simulink model "Biomech_Project_LQR_cleanup"  (R2017a)
settings: Solver=ode45  StartTime=0.0  StopTime=10  MaxStep=1e-3  RelTol=1e-4  AbsTol=1e-6  EnableMultiTasking=on
values from neighbouring files (symbols this model uses):
  g = 9.81    [Biomech_Project_LQR_param.mat]
  K = [0.0235570993622  0.453677279991  -0.304744102928; 0.280809210373  -0.335573491599  -0.504535045423]    [Biomech_Project_LQR_param.mat]    (also in QRABK_LQR_controller.mat)
  L = 0.2    [Biomech_Project_LQR_param.mat]
  l0 = 0.2    [Biomech_Project_LQR_param.mat]
  m = 6    [Biomech_Project_LQR_param.mat]
  x0 = []    [AnimQUAD.m]    (also in Biomech_Project_LQR_param.mat = 0)
  xrb0 = 0.130612869685    [Biomech_Project_LQR_param.mat]
  xrf0 = -0.273446372372    [Biomech_Project_LQR_param.mat]
  y0 = 1    [Biomech_Project_LQR_param.mat]
  yrb0 = 0.187577786922    [Biomech_Project_LQR_param.mat]
  yrf0 = 0.186025886331    [Biomech_Project_LQR_param.mat]
libraries: simulink_extras x4
settings Model: Creator=hgeyer  LastModifiedBy=shawn
settings DataIOCC: SaveFormat=Array  SignalLoggingSaveFormat=ModelDataLogs
settings OptimizationCC: ExpressionDepthLimit=2147483647  LifeSpan=inf
settings DebuggingCC: UnderspecifiedInitializationDetection=Classic  MergeDetectMultiDrivingBlocksExec=none  SolverPrmCheckMsg=warning  FcnCallInpInsideContextMsg=warning  AllowSymbolicDim=off  StateNameClashWarn=warning  SFUnexpectedBacktrackingDiag=warning  SFNoUnconditionalDefaultTransitionDiag=warning  SFExecutionAtInitializationDiag=none
settings HardwareCC: ProdBitPerPointer=32  ProdBitPerSizeT=32  ProdBitPerPtrDiffT=32  ProdLargestAtomicFloat=None  ProdIntDivRoundTo=Undefined  ProdEndianess=Unspecified  ProdWordSize=32  ProdHWDeviceType=32-bit Generic
settings ModelReferenceCC: PropagateSignalLabelsOutOfModel=off
settings GRTTargetCC: TargetLangStandard=C89/C90 (ANSI)  GeneratePreprocessorConditionals=Disable all
settings ConfigComp: CovMetricSettings=dw  CovHtmlReporting=on  CovSaveCumulativeToWorkspaceVar=on  CovSaveSingleToWorkspaceVar=on  CovExternalEMLEnable=off

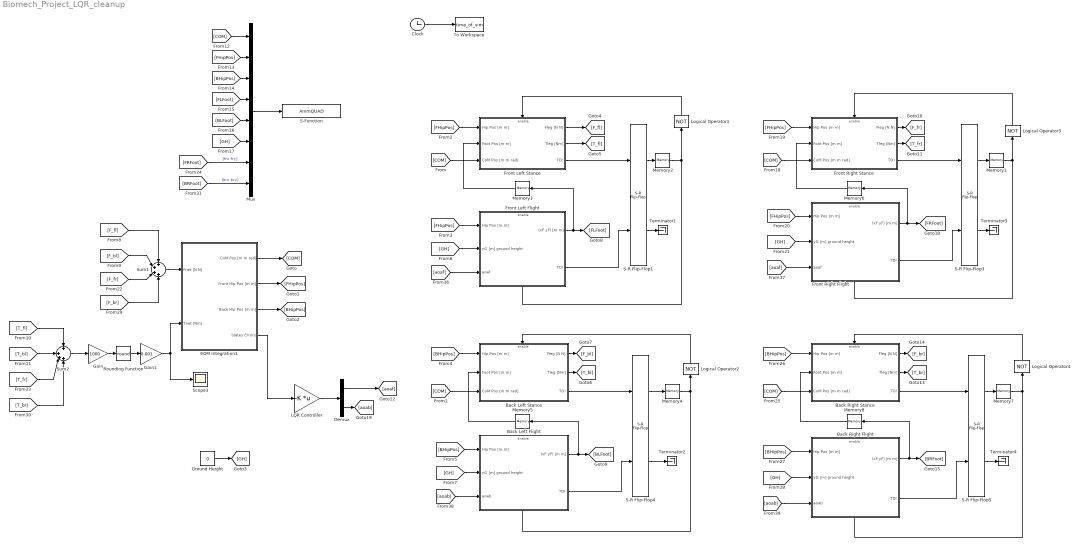
== system Biomech_Project_LQR_cleanup ==
  Back Left Flight : Subsystem
  Back Left Stance : Subsystem
  Back Right Flight : Subsystem
  Back Right Stance : Subsystem
  Clock : Clock
      settings: Decimation=100
  Demux : Demux  Outputs=2
  EOM Integration1 : Subsystem
  Front Left Flight : Subsystem
  Front Left Stance : Subsystem
  Front Right Flight : Subsystem
  Front Right Stance : Subsystem
  Gain : Gain  Gain=1000
  Gain1 : Gain  Gain=0.001
  Ground Height : Constant  Value=0
  LQR Controller : Gain  Gain=-K  Multiplication=Matrix(K*u)
  Logical Operator{1..4} (4 alike) : Logic  Operator=NOT  AllPortsSameDT=off  OutDataTypeStr=boolean
  Memory{1..2,4,7} (4 alike) : Memory  X0=1
  Memory3 : Memory  X0=[(x0 - xrf0) (y0 - yrf0) ]
  Memory5 : Memory  X0=[(x0 - xrb0) (y0 - yrb0)]
  Memory6 : Memory  X0=[(x0 - xrf0) (y0 - yrf0) ]
  Memory8 : Memory  X0=[(x0 - xrb0) (y0 - yrb0)]
  Mux : Mux  Inputs=8
  Rounding Function : Rounding  Operator=round
  S-Function : S-Function  FunctionName=AnimQUAD  Parameters=0.005  SFunctionDeploymentMode=off  EnableBusSupport=off
  S-R Flip-Flop{1,3..5} (4 alike) : simulink_extras/Flip Flops/S-R Flip-Flop  initial_condition=1
  Scope3 : Scope
  Sum1 : Sum  Inputs=++++
  Sum2 : Sum  Inputs=+|+++
  Terminator{1..4} (4 alike) : Terminator
  To Workspace : ToWorkspace  VariableName=time_of_sim  SampleTime=-1
      settings: MaxDataPoints=1
  wires:
  S-R Flip-Flop1/1 -> Memory2/1
  Memory2/1 -> Front Left Flight/Enable, Logical Operator1/1
  Logical Operator1/1 -> Front Left Stance/Enable
  S-R Flip-Flop1/2 -> Terminator1/1
  Front Left Flight/1((xF yF) [m m]) -> Memory3/1, [FLFoot]
  Memory3/1 -> Front Left Stance/2(Foot Pos [m m])
  Back Left Stance/3(TO!) -> S-R Flip-Flop4/1
  S-R Flip-Flop4/1 -> Memory4/1
  Back Left Flight/2(TD!) -> S-R Flip-Flop4/2
  Memory4/1 -> Back Left Flight/Enable, Logical Operator2/1
  Logical Operator2/1 -> Back Left Stance/Enable
  S-R Flip-Flop4/2 -> Terminator2/1
  [GH] -> Back Left Flight/2(yG [m] ground height)
  Back Left Flight/1((xF yF) [m m]) -> [BLFoot], Memory5/1
  Memory5/1 -> Back Left Stance/2(Foot Pos [m m])
  Ground Height/1 -> [GH]
  [GH] -> Front Left Flight/2(yG [m] ground height)
  Front Left Stance/1(Fleg [N N]) -> [F_fl]
  Front Left Stance/2(Tleg [Nm]) -> [T_fl]
  Back Left Stance/1(Fleg [N N]) -> [F_bl]
  Back Left Stance/2(Tleg [Nm]) -> [T_bl]
  [F_fl] -> Sum1/1
  [F_bl] -> Sum1/2
  [T_fl] -> Sum2/1
  [T_bl] -> Sum2/2
  Sum1/1 -> EOM Integration1/1(Fnet [N N])
  EOM Integration1/1(CoM Pos [m m rad]) -> [COM]
  EOM Integration1/2(Front Hip Pos [m m]) -> [FHipPos]
  EOM Integration1/3(Back Hip Pos [m m]) -> [BHipPos]
  [FHipPos] -> Front Left Stance/1(Hip Pos [m m])
  [FHipPos] -> Front Left Flight/1(Hip Pos [m m])
  [BHipPos] -> Back Left Stance/1(Hip Pos [m m])
  [BHipPos] -> Back Left Flight/1(Hip Pos [m m])
  [COM] -> Front Left Stance/3(CoM Pos [m m rad])
  [COM] -> Back Left Stance/3(CoM Pos [m m rad])
  Sum2/1 -> Gain/1
  Gain1/1 -> Scope3/1, EOM Integration1/2(Tnet [Nm])
  Gain/1 -> Rounding Function/1
  Rounding Function/1 -> Gain1/1
  Mux/1 -> S-Function/1
  [COM] -> Mux/1
  [FHipPos] -> Mux/2
  [BHipPos] -> Mux/3
  [FLFoot] -> Mux/4
  [BLFoot] -> Mux/5
  [GH] -> Mux/6
  [FRFoot] -> Mux/7  "[frx fry]"
  [BRFoot] -> Mux/8  "[brx bry]"
  S-R Flip-Flop3/1 -> Memory1/1
  Memory1/1 -> Front Right Flight/Enable, Logical Operator3/1
  Logical Operator3/1 -> Front Right Stance/Enable
  S-R Flip-Flop3/2 -> Terminator3/1
  Front Right Flight/1((xF yF) [m m]) -> [FRFoot], Memory6/1
  Memory6/1 -> Front Right Stance/2(Foot Pos [m m])
  [GH] -> Front Right Flight/2(yG [m] ground height)
  Front Right Stance/1(Fleg [N N]) -> [F_fr]
  Front Right Stance/2(Tleg [Nm]) -> [T_fr]
  [FHipPos] -> Front Right Stance/1(Hip Pos [m m])
  [FHipPos] -> Front Right Flight/1(Hip Pos [m m])
  [COM] -> Front Right Stance/3(CoM Pos [m m rad])
  [F_fr] -> Sum1/3
  [T_fr] -> Sum2/3
  Back Right Stance/3(TO!) -> S-R Flip-Flop5/1
  S-R Flip-Flop5/1 -> Memory7/1
  Back Right Flight/2(TD!) -> S-R Flip-Flop5/2
  Memory7/1 -> Back Right Flight/Enable, Logical Operator4/1
  Logical Operator4/1 -> Back Right Stance/Enable
  S-R Flip-Flop5/2 -> Terminator4/1
  [GH] -> Back Right Flight/2(yG [m] ground height)
  Back Right Flight/1((xF yF) [m m]) -> [BRFoot], Memory8/1
  Memory8/1 -> Back Right Stance/2(Foot Pos [m m])
  Back Right Stance/1(Fleg [N N]) -> [F_br]
  Back Right Stance/2(Tleg [Nm]) -> [T_br]
  [BHipPos] -> Back Right Stance/1(Hip Pos [m m])
  [BHipPos] -> Back Right Flight/1(Hip Pos [m m])
  [COM] -> Back Right Stance/3(CoM Pos [m m rad])
  [F_br] -> Sum1/4
  [T_br] -> Sum2/4
  Clock/1 -> To Workspace/1
  Front Right Stance/3(TO!) -> S-R Flip-Flop3/1
  Front Right Flight/2(TD!) -> S-R Flip-Flop3/2
  Front Left Stance/3(TO!) -> S-R Flip-Flop1/1
  Front Left Flight/2(TD!) -> S-R Flip-Flop1/2
  EOM Integration1/4(States Errors) -> LQR Controller/1
  LQR Controller/1 -> Demux/1
  Demux/1 -> [aoaf]
  Demux/2 -> [aoab]
  [aoaf] -> Front Left Flight/3("aoaf ")
  [aoaf] -> Front Right Flight/3("aoaf ")
  [aoab] -> Back Left Flight/3(aoab)
  [aoab] -> Back Right Flight/3(aoab)

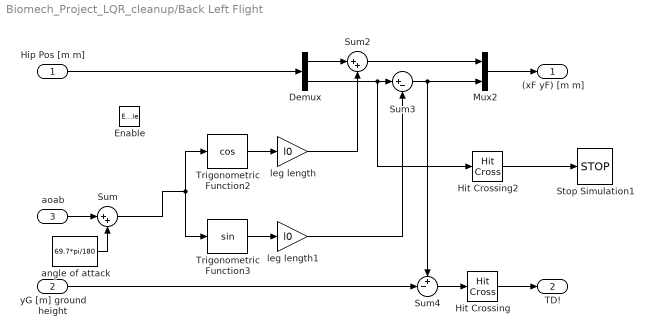
== system Biomech_Project_LQR_cleanup/Back Left Flight ==
  Hip Pos [m m] : Inport
  yG [m] ground height : Inport  Port=2
  aoab : Inport  Port=3
  Enable : EnablePort  StatesWhenEnabling=reset
  Demux : Demux  Outputs=2
  Hit Crossing : HitCross  HitCrossingDirection=falling
  Hit Crossing2 : HitCross  HitCrossingOffset=-1  HitCrossingDirection=falling
  Mux2 : Mux  Inputs=2
  Stop Simulation1 : Stop
  Sum : Sum  Inputs=|++
  Sum2 : Sum  Inputs=|++
  Sum3 : Sum  Inputs=|+-
  Sum4 : Sum  Inputs=+-|
  Trigonometric Function2 : Trigonometry  Operator=cos
  Trigonometric Function3 : Trigonometry
  angle of attack : Constant  Value=69.7*pi/180
  leg length : Gain  Gain=l0
  leg length1 : Gain  Gain=l0
  (xF yF) [m m] : Outport  InitialOutput=[0 0]
      settings: AttributesFormatString=%<OutputWhenDisabled>
  TD! : Outport  Port=2  OutputWhenDisabled=reset  InitialOutput=0
      settings: AttributesFormatString=%<OutputWhenDisabled>
  wires:
  Demux/2 -> Hit Crossing2/1, Sum3/1
  Demux/1 -> Sum2/1
  Sum/1 -> Trigonometric Function3/1, Trigonometric Function2/1
  Trigonometric Function2/1 -> leg length/1
  Trigonometric Function3/1 -> leg length1/1
  Hip Pos [m m]/1 -> Demux/1
  leg length/1 -> Sum2/2
  leg length1/1 -> Sum3/2
  Sum3/1 -> Mux2/2, Sum4/1
  Sum2/1 -> Mux2/1
  Mux2/1 -> (xF yF) [m m]/1
  yG [m] ground height/1 -> Sum4/2
  Sum4/1 -> Hit Crossing/1
  Hit Crossing2/1 -> Stop Simulation1/1
  Hit Crossing/1 -> TD!/1
  aoab/1 -> Sum/1
  angle of attack/1 -> Sum/2

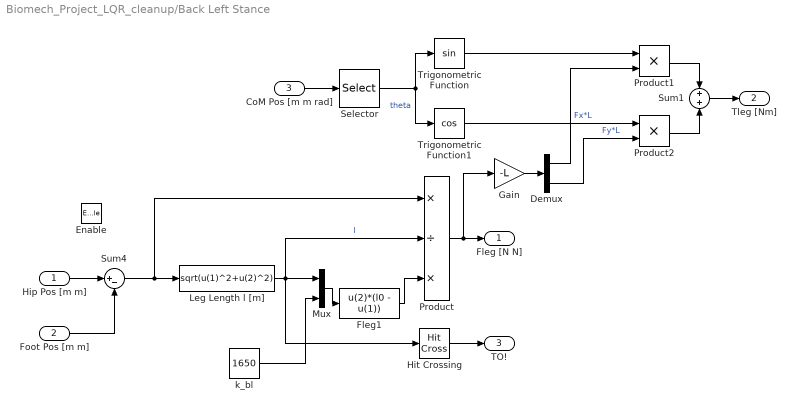
== system Biomech_Project_LQR_cleanup/Back Left Stance ==
  Hip Pos [m m] : Inport
  Foot Pos [m m] : Inport  Port=2
  CoM Pos [m m rad] : Inport  Port=3
  Enable : EnablePort  StatesWhenEnabling=reset
  Demux : Demux  Outputs=2
  Fleg1 : Fcn  Expr=u(2)*(l0 - u(1))
  Gain : Gain  Gain=-L
  Hit Crossing : HitCross  HitCrossingOffset=l0  HitCrossingDirection=rising
  Leg Length l [m] : Fcn  Expr=sqrt(u(1)^2+u(2)^2)
  Mux : Mux  Inputs=2
  Product : Product  Inputs=*/*
  Product1 : Product
  Product2 : Product
  Selector : Selector  InputPortWidth=3  IndexOptions=Index vector (dialog)  Indices=[3]  OutputSizes=1
  Sum1 : Sum  Inputs=+|+
  Sum4 : Sum  Inputs=|+-
  Trigonometric Function : Trigonometry
  Trigonometric Function1 : Trigonometry  Operator=cos
  k_bl : Constant  Value=1650
  Fleg [N N] : Outport  OutputWhenDisabled=reset  InitialOutput=[0 0]
      settings: AttributesFormatString=%<OutputWhenDisabled>
  Tleg [Nm] : Outport  Port=2  OutputWhenDisabled=reset  InitialOutput=[0]
      settings: AttributesFormatString=%<OutputWhenDisabled>
  TO! : Outport  Port=3  OutputWhenDisabled=reset  InitialOutput=[0]
      settings: AttributesFormatString=%<OutputWhenDisabled>
  wires:
  Sum1/1 -> Tleg [Nm]/1
  Product1/1 -> Sum1/1
  Product2/1 -> Sum1/2
  Gain/1 -> Demux/1
  Demux/2 -> Product2/2  "Fy*L"
  Demux/1 -> Product1/2  "Fx*L"
  Trigonometric Function/1 -> Product1/1
  Trigonometric Function1/1 -> Product2/1
  Selector/1 -> Trigonometric Function/1, Trigonometric Function1/1  "theta"
  CoM Pos [m m rad]/1 -> Selector/1
  Foot Pos [m m]/1 -> Sum4/2
  Hip Pos [m m]/1 -> Sum4/1
  Hit Crossing/1 -> TO!/1
  Product/1 -> Fleg [N N]/1, Gain/1
  Fleg1/1 -> Product/3
  Leg Length l [m]/1 -> Hit Crossing/1, Mux/1, Product/2  "l"
  Sum4/1 -> Leg Length l [m]/1, Product/1
  Mux/1 -> Fleg1/1
  k_bl/1 -> Mux/2

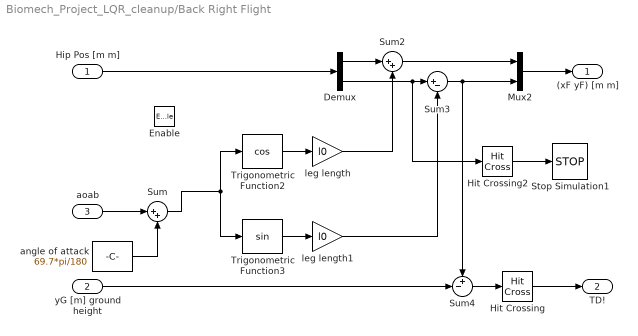
== system Biomech_Project_LQR_cleanup/Back Right Flight ==
  Hip Pos [m m] : Inport
  yG [m] ground height : Inport  Port=2
  aoab : Inport  Port=3
  Enable : EnablePort  StatesWhenEnabling=reset
  Demux : Demux  Outputs=2
  Hit Crossing : HitCross  HitCrossingDirection=falling
  Hit Crossing2 : HitCross  HitCrossingOffset=-1  HitCrossingDirection=falling
  Mux2 : Mux  Inputs=2
  Stop Simulation1 : Stop
  Sum : Sum  Inputs=|++
  Sum2 : Sum  Inputs=|++
  Sum3 : Sum  Inputs=|+-
  Sum4 : Sum  Inputs=+-|
  Trigonometric Function2 : Trigonometry  Operator=cos
  Trigonometric Function3 : Trigonometry
  angle of attack : Constant  Value=69.7*pi/180
  leg length : Gain  Gain=l0
  leg length1 : Gain  Gain=l0
  (xF yF) [m m] : Outport  InitialOutput=[0 0]
      settings: AttributesFormatString=%<OutputWhenDisabled>
  TD! : Outport  Port=2  OutputWhenDisabled=reset  InitialOutput=0
      settings: AttributesFormatString=%<OutputWhenDisabled>
  wires:
  Sum4/1 -> Hit Crossing/1
  yG [m] ground height/1 -> Sum4/2
  Mux2/1 -> (xF yF) [m m]/1
  Sum2/1 -> Mux2/1
  Sum3/1 -> Sum4/1, Mux2/2
  leg length1/1 -> Sum3/2
  leg length/1 -> Sum2/2
  Hip Pos [m m]/1 -> Demux/1
  Trigonometric Function3/1 -> leg length1/1
  Trigonometric Function2/1 -> leg length/1
  Sum/1 -> Trigonometric Function2/1, Trigonometric Function3/1
  Demux/1 -> Sum2/1
  Demux/2 -> Hit Crossing2/1, Sum3/1
  Hit Crossing2/1 -> Stop Simulation1/1
  aoab/1 -> Sum/1
  angle of attack/1 -> Sum/2
  Hit Crossing/1 -> TD!/1

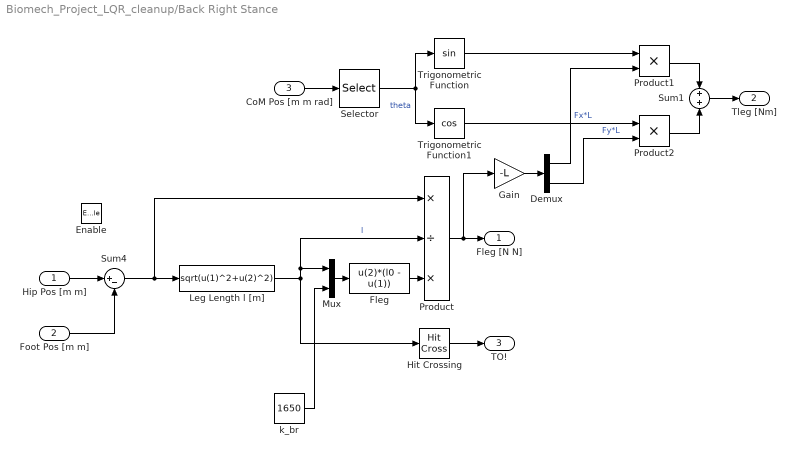
== system Biomech_Project_LQR_cleanup/Back Right Stance ==
  Hip Pos [m m] : Inport
  Foot Pos [m m] : Inport  Port=2
  CoM Pos [m m rad] : Inport  Port=3
  Enable : EnablePort  StatesWhenEnabling=reset
  Demux : Demux  Outputs=2
  Fleg : Fcn  Expr=u(2)*(l0 - u(1))
  Gain : Gain  Gain=-L
  Hit Crossing : HitCross  HitCrossingOffset=l0  HitCrossingDirection=rising
  Leg Length l [m] : Fcn  Expr=sqrt(u(1)^2+u(2)^2)
  Mux : Mux  Inputs=2
  Product : Product  Inputs=*/*
  Product1 : Product
  Product2 : Product
  Selector : Selector  InputPortWidth=3  IndexOptions=Index vector (dialog)  Indices=[3]  OutputSizes=1
  Sum1 : Sum  Inputs=+|+
  Sum4 : Sum  Inputs=|+-
  Trigonometric Function : Trigonometry
  Trigonometric Function1 : Trigonometry  Operator=cos
  k_br : Constant  Value=1650
  Fleg [N N] : Outport  OutputWhenDisabled=reset  InitialOutput=[0 0]
      settings: AttributesFormatString=%<OutputWhenDisabled>
  Tleg [Nm] : Outport  Port=2  OutputWhenDisabled=reset  InitialOutput=[0]
      settings: AttributesFormatString=%<OutputWhenDisabled>
  TO! : Outport  Port=3  OutputWhenDisabled=reset  InitialOutput=[0]
      settings: AttributesFormatString=%<OutputWhenDisabled>
  wires:
  Sum1/1 -> Tleg [Nm]/1
  Product1/1 -> Sum1/1
  Product2/1 -> Sum1/2
  Gain/1 -> Demux/1
  Demux/2 -> Product2/2  "Fy*L"
  Demux/1 -> Product1/2  "Fx*L"
  Trigonometric Function/1 -> Product1/1
  Trigonometric Function1/1 -> Product2/1
  Selector/1 -> Trigonometric Function/1, Trigonometric Function1/1  "theta"
  CoM Pos [m m rad]/1 -> Selector/1
  Foot Pos [m m]/1 -> Sum4/2
  Hip Pos [m m]/1 -> Sum4/1
  Hit Crossing/1 -> TO!/1
  Product/1 -> Fleg [N N]/1, Gain/1
  Fleg/1 -> Product/3
  Leg Length l [m]/1 -> Mux/1, Product/2, Hit Crossing/1  "l"
  Sum4/1 -> Leg Length l [m]/1, Product/1
  Mux/1 -> Fleg/1
  k_br/1 -> Mux/2

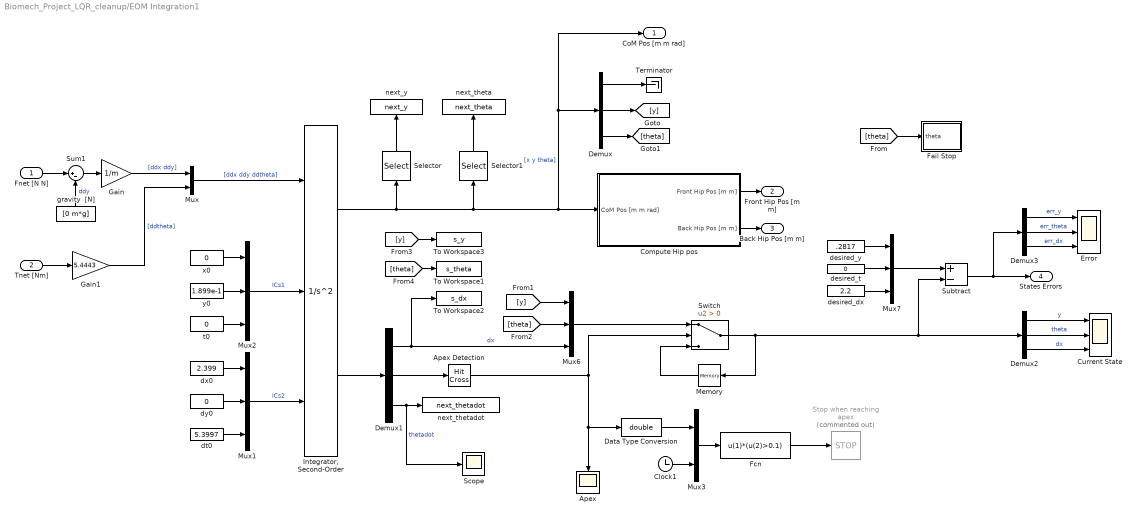
== system Biomech_Project_LQR_cleanup/EOM Integration1 ==
  Fnet [N N] : Inport
  Tnet [Nm] : Inport  Port=2
  Apex : Scope
  Apex Detection : HitCross  HitCrossingOffset=0.0001  HitCrossingDirection=falling
  Clock1 : Clock
  Compute Hip pos : Subsystem
  Current State : Scope  NumInputPorts=3
  Data Type Conversion : DataTypeConversion  OutDataTypeStr=double
  Demux{,1..3} (4 alike) : Demux  Outputs=3
  Error : Scope  NumInputPorts=3
  Fail Stop : Subsystem
  Fcn : Fcn  Expr=u(1)*(u(2)>0.1)
  Gain : Gain  Gain=1/m
  Gain1 : Gain  Gain=5.4443
  "Integrator, Second-Order" : SecondOrderIntegrator  ICSourceX=external  ICSourceDXDT=external
  Memory : Memory  X0=[0.2817 0 2.2]
  Mux : Mux  Inputs=2
  Mux{1..2,6..7} (4 alike) : Mux  Inputs=3
  Mux3 : Mux  Inputs=2
  Scope : Scope
  Selector : Selector  InputPortWidth=3  IndexOptions=Index vector (dialog)  Indices=[2]  OutputSizes=1
  Selector1 : Selector  InputPortWidth=3  IndexOptions=Index vector (dialog)  Indices=[3]  OutputSizes=1
  Stop when reaching apex : Stop  Commented=on
  Subtract : Sum  Inputs=+-
  Sum1 : Sum  Inputs=|+-
  Switch : Switch  Criteria=u2 > Threshold
  Terminator : Terminator
  To Workspace1 : ToWorkspace  VariableName=s_theta  SampleTime=-1
      settings: Save2DSignal=2-D array (concatenate along first dimension)
  To Workspace2 : ToWorkspace  VariableName=s_dx  SampleTime=-1
      settings: Save2DSignal=2-D array (concatenate along first dimension)
  To Workspace3 : ToWorkspace  VariableName=s_y  SampleTime=-1
      settings: Save2DSignal=2-D array (concatenate along first dimension)
  "desired_dx " : Constant  Value=2.2
  desired_t : Constant  Value=0
  desired_y : Constant  Value=.2817
  dt0 : Constant  Value=5.3997
  dx0 : Constant  Value=2.399
  dy0 : Constant  Value=0
  gravity  [N] : Constant  Value=[0 m*g]
  next_theta : ToWorkspace  VariableName=next_theta  SampleTime=-1
      settings: MaxDataPoints=1
  next_thetadot : ToWorkspace  VariableName=next_thetadot  SampleTime=-1
      settings: MaxDataPoints=1
  next_y : ToWorkspace  VariableName=next_y  SampleTime=-1
      settings: MaxDataPoints=1
  t0 : Constant  Value=0
  x0 : Constant  Value=0
  y0 : Constant  Value=1.899e-1
  CoM Pos [m m rad] : Outport
  Front Hip Pos [m m] : Outport  Port=2
  Back Hip Pos [m m] : Outport  Port=3
  States Errors : Outport  Port=4
  wires:
  Compute Hip pos/1(Front Hip Pos [m m]) -> Front Hip Pos [m m]/1
  "Integrator, Second-Order"/1 -> Compute Hip pos/1(CoM Pos [m m rad]), CoM Pos [m m rad]/1, Demux/1, Selector1/1, Selector/1  "[x y theta]"
  Tnet [Nm]/1 -> Gain1/1
  Gain1/1 -> Mux/2  "[ddtheta]"
  Mux/1 -> "Integrator, Second-Order"/1  "[ddx ddy ddtheta]"
  Fnet [N N]/1 -> Sum1/1
  Gain/1 -> Mux/1  "[ddx ddy]"
  gravity  [N]/1 -> Sum1/2  "ddy"
  Sum1/1 -> Gain/1
  Compute Hip pos/2(Back Hip Pos [m m]) -> Back Hip Pos [m m]/1
  dx0/1 -> Mux1/1
  dy0/1 -> Mux1/2
  dt0/1 -> Mux1/3
  Demux/3 -> [theta]
  Demux/1 -> Terminator/1
  Demux/2 -> [y]
  Apex Detection/1 -> Switch/2, Apex/1, Data Type Conversion/1
  "Integrator, Second-Order"/2 -> Demux1/1
  x0/1 -> Mux2/1
  y0/1 -> Mux2/2
  t0/1 -> Mux2/3
  Demux1/2 -> Apex Detection/1
  Demux1/1 -> To Workspace2/1, Mux6/3  "dx"
  Clock1/1 -> Mux3/2
  Mux3/1 -> Fcn/1
  Data Type Conversion/1 -> Mux3/1
  Selector/1 -> next_y/1
  Fcn/1 -> Stop when reaching apex/1
  Selector1/1 -> next_theta/1
  Mux1/1 -> "Integrator, Second-Order"/3  "ICs2"
  Mux2/1 -> "Integrator, Second-Order"/2  "ICs1"
  Mux6/1 -> Switch/1
  Switch/1 -> Demux2/1, Subtract/2, Memory/1
  Memory/1 -> Switch/3
  desired_y/1 -> Mux7/1
  desired_t/1 -> Mux7/2
  "desired_dx "/1 -> Mux7/3
  Subtract/1 -> Demux3/1, States Errors/1
  Mux7/1 -> Subtract/1
  Demux1/3 -> Scope/1, next_thetadot/1  "thetadot"
  [theta] -> Fail Stop/1(theta)
  [y] -> Mux6/1
  [theta] -> Mux6/2
  Demux2/1 -> Current State/1  "y"
  Demux2/2 -> Current State/2  "theta"
  Demux2/3 -> Current State/3  "dx"
  Demux3/3 -> Error/3  "err_dx"
  Demux3/2 -> Error/2  "err_theta"
  Demux3/1 -> Error/1  "err_y"
  [y] -> To Workspace3/1
  [theta] -> To Workspace1/1

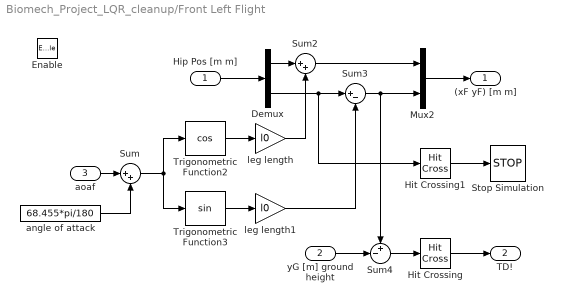
== system Biomech_Project_LQR_cleanup/Front Left Flight ==
  Hip Pos [m m] : Inport
  yG [m] ground height : Inport  Port=2
  "aoaf " : Inport  Port=3
  Enable : EnablePort  StatesWhenEnabling=reset
  Demux : Demux  Outputs=2
  Hit Crossing : HitCross  HitCrossingDirection=falling
  Hit Crossing1 : HitCross  HitCrossingOffset=-1  HitCrossingDirection=falling
  Mux2 : Mux  Inputs=2
  Stop Simulation : Stop
  Sum : Sum  Inputs=|++
  Sum2 : Sum  Inputs=|++
  Sum3 : Sum  Inputs=|+-
  Sum4 : Sum  Inputs=+-|
  Trigonometric Function2 : Trigonometry  Operator=cos
  Trigonometric Function3 : Trigonometry
  angle of attack : Constant  Value=68.455*pi/180
  leg length : Gain  Gain=l0
  leg length1 : Gain  Gain=l0
  (xF yF) [m m] : Outport  InitialOutput=[0 0]
      settings: AttributesFormatString=%<OutputWhenDisabled>
  TD! : Outport  Port=2  OutputWhenDisabled=reset  InitialOutput=0
      settings: AttributesFormatString=%<OutputWhenDisabled>
  wires:
  Hit Crossing1/1 -> Stop Simulation/1
  Sum4/1 -> Hit Crossing/1
  yG [m] ground height/1 -> Sum4/2
  Mux2/1 -> (xF yF) [m m]/1
  Sum2/1 -> Mux2/1
  Sum3/1 -> Mux2/2, Sum4/1
  leg length1/1 -> Sum3/2
  leg length/1 -> Sum2/2
  Hip Pos [m m]/1 -> Demux/1
  Trigonometric Function3/1 -> leg length1/1
  Trigonometric Function2/1 -> leg length/1
  Sum/1 -> Trigonometric Function2/1, Trigonometric Function3/1
  Demux/1 -> Sum2/1
  Demux/2 -> Hit Crossing1/1, Sum3/1
  Hit Crossing/1 -> TD!/1
  "aoaf "/1 -> Sum/1
  angle of attack/1 -> Sum/2

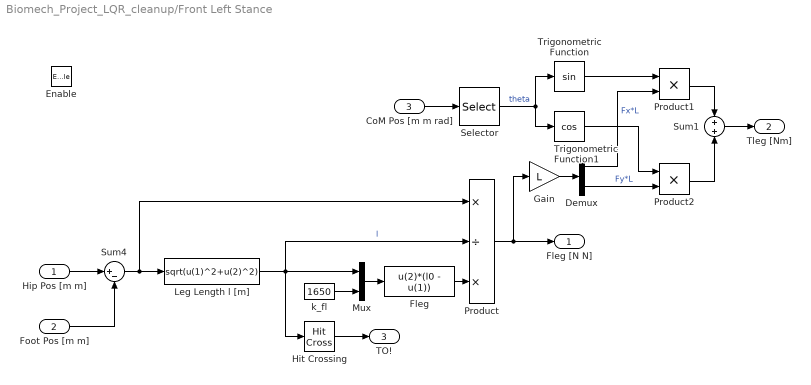
== system Biomech_Project_LQR_cleanup/Front Left Stance ==
  Hip Pos [m m] : Inport
  Foot Pos [m m] : Inport  Port=2
  CoM Pos [m m rad] : Inport  Port=3
  Enable : EnablePort  StatesWhenEnabling=reset
  Demux : Demux  Outputs=2
  Fleg : Fcn  Expr=u(2)*(l0 - u(1))
  Gain : Gain  Gain=L
  Hit Crossing : HitCross  HitCrossingOffset=l0  HitCrossingDirection=rising
  Leg Length l [m] : Fcn  Expr=sqrt(u(1)^2+u(2)^2)
  Mux : Mux  Inputs=2
  Product : Product  Inputs=*/*
  Product1 : Product
  Product2 : Product
  Selector : Selector  InputPortWidth=3  IndexOptions=Index vector (dialog)  Indices=[3]  OutputSizes=1
  Sum1 : Sum  Inputs=+|+
  Sum4 : Sum  Inputs=|+-
  Trigonometric Function : Trigonometry
  Trigonometric Function1 : Trigonometry  Operator=cos
  k_fl : Constant  Value=1650
  Fleg [N N] : Outport  OutputWhenDisabled=reset  InitialOutput=[0 0]
      settings: AttributesFormatString=%<OutputWhenDisabled>
  Tleg [Nm] : Outport  Port=2  OutputWhenDisabled=reset  InitialOutput=[0]
      settings: AttributesFormatString=%<OutputWhenDisabled>
  TO! : Outport  Port=3  OutputWhenDisabled=reset  InitialOutput=[0]
      settings: AttributesFormatString=%<OutputWhenDisabled>
  wires:
  Sum4/1 -> Product/1, Leg Length l [m]/1
  Leg Length l [m]/1 -> Hit Crossing/1, Mux/1, Product/2  "l"
  Fleg/1 -> Product/3
  Product/1 -> Gain/1, Fleg [N N]/1
  Hit Crossing/1 -> TO!/1
  Hip Pos [m m]/1 -> Sum4/1
  Foot Pos [m m]/1 -> Sum4/2
  CoM Pos [m m rad]/1 -> Selector/1
  Selector/1 -> Trigonometric Function/1, Trigonometric Function1/1  "theta"
  Trigonometric Function1/1 -> Product2/1
  Trigonometric Function/1 -> Product1/1
  Demux/1 -> Product1/2  "Fx*L"
  Demux/2 -> Product2/2  "Fy*L"
  Gain/1 -> Demux/1
  Product2/1 -> Sum1/2
  Product1/1 -> Sum1/1
  Sum1/1 -> Tleg [Nm]/1
  Mux/1 -> Fleg/1
  k_fl/1 -> Mux/2

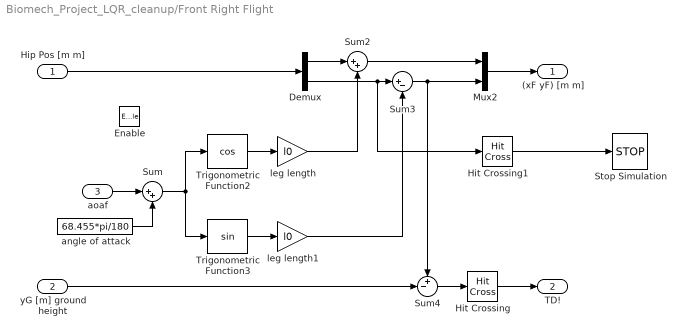
== system Biomech_Project_LQR_cleanup/Front Right Flight ==
  Hip Pos [m m] : Inport
  yG [m] ground height : Inport  Port=2
  "aoaf " : Inport  Port=3
  Enable : EnablePort  StatesWhenEnabling=reset
  Demux : Demux  Outputs=2
  Hit Crossing : HitCross  HitCrossingDirection=falling
  Hit Crossing1 : HitCross  HitCrossingOffset=-1  HitCrossingDirection=falling
  Mux2 : Mux  Inputs=2
  Stop Simulation : Stop
  Sum : Sum  Inputs=|++
  Sum2 : Sum  Inputs=|++
  Sum3 : Sum  Inputs=|+-
  Sum4 : Sum  Inputs=+-|
  Trigonometric Function2 : Trigonometry  Operator=cos
  Trigonometric Function3 : Trigonometry
  angle of attack : Constant  Value=68.455*pi/180
  leg length : Gain  Gain=l0
  leg length1 : Gain  Gain=l0
  (xF yF) [m m] : Outport  InitialOutput=[0 0]
      settings: AttributesFormatString=%<OutputWhenDisabled>
  TD! : Outport  Port=2  OutputWhenDisabled=reset  InitialOutput=0
      settings: AttributesFormatString=%<OutputWhenDisabled>
  wires:
  Demux/2 -> Hit Crossing1/1, Sum3/1
  Demux/1 -> Sum2/1
  Sum/1 -> Trigonometric Function3/1, Trigonometric Function2/1
  Trigonometric Function2/1 -> leg length/1
  Trigonometric Function3/1 -> leg length1/1
  Hip Pos [m m]/1 -> Demux/1
  leg length/1 -> Sum2/2
  leg length1/1 -> Sum3/2
  Sum3/1 -> Mux2/2, Sum4/1
  Sum2/1 -> Mux2/1
  Mux2/1 -> (xF yF) [m m]/1
  yG [m] ground height/1 -> Sum4/2
  Sum4/1 -> Hit Crossing/1
  Hit Crossing1/1 -> Stop Simulation/1
  Hit Crossing/1 -> TD!/1
  "aoaf "/1 -> Sum/1
  angle of attack/1 -> Sum/2

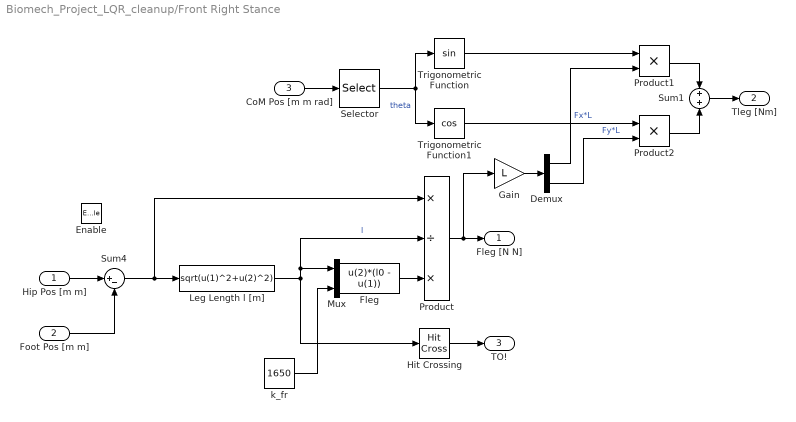
== system Biomech_Project_LQR_cleanup/Front Right Stance ==
  Hip Pos [m m] : Inport
  Foot Pos [m m] : Inport  Port=2
  CoM Pos [m m rad] : Inport  Port=3
  Enable : EnablePort  StatesWhenEnabling=reset
  Demux : Demux  Outputs=2
  Fleg : Fcn  Expr=u(2)*(l0 - u(1))
  Gain : Gain  Gain=L
  Hit Crossing : HitCross  HitCrossingOffset=l0  HitCrossingDirection=rising
  Leg Length l [m] : Fcn  Expr=sqrt(u(1)^2+u(2)^2)
  Mux : Mux  Inputs=2
  Product : Product  Inputs=*/*
  Product1 : Product
  Product2 : Product
  Selector : Selector  InputPortWidth=3  IndexOptions=Index vector (dialog)  Indices=[3]  OutputSizes=1
  Sum1 : Sum  Inputs=+|+
  Sum4 : Sum  Inputs=|+-
  Trigonometric Function : Trigonometry
  Trigonometric Function1 : Trigonometry  Operator=cos
  k_fr : Constant  Value=1650
  Fleg [N N] : Outport  OutputWhenDisabled=reset  InitialOutput=[0 0]
      settings: AttributesFormatString=%<OutputWhenDisabled>
  Tleg [Nm] : Outport  Port=2  OutputWhenDisabled=reset  InitialOutput=[0]
      settings: AttributesFormatString=%<OutputWhenDisabled>
  TO! : Outport  Port=3  OutputWhenDisabled=reset  InitialOutput=[0]
      settings: AttributesFormatString=%<OutputWhenDisabled>
  wires:
  Sum4/1 -> Product/1, Leg Length l [m]/1
  Leg Length l [m]/1 -> Mux/1, Product/2, Hit Crossing/1  "l"
  Fleg/1 -> Product/3
  Product/1 -> Gain/1, Fleg [N N]/1
  Hit Crossing/1 -> TO!/1
  Hip Pos [m m]/1 -> Sum4/1
  Foot Pos [m m]/1 -> Sum4/2
  CoM Pos [m m rad]/1 -> Selector/1
  Selector/1 -> Trigonometric Function1/1, Trigonometric Function/1  "theta"
  Trigonometric Function1/1 -> Product2/1
  Trigonometric Function/1 -> Product1/1
  Demux/1 -> Product1/2  "Fx*L"
  Demux/2 -> Product2/2  "Fy*L"
  Gain/1 -> Demux/1
  Product2/1 -> Sum1/2
  Product1/1 -> Sum1/1
  Sum1/1 -> Tleg [Nm]/1
  Mux/1 -> Fleg/1
  k_fr/1 -> Mux/2

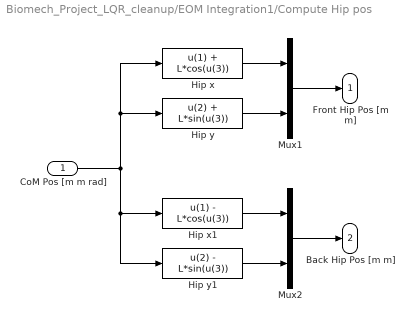
== system Biomech_Project_LQR_cleanup/EOM Integration1/Compute Hip pos ==
  CoM Pos [m m rad] : Inport
  Hip x : Fcn  Expr=u(1) + L*cos(u(3))
  Hip x1 : Fcn  Expr=u(1) - L*cos(u(3))
  Hip y : Fcn  Expr=u(2) + L*sin(u(3))
  Hip y1 : Fcn  Expr=u(2) - L*sin(u(3))
  Mux1 : Mux  Inputs=2
  Mux2 : Mux  Inputs=2
  Front Hip Pos [m m] : Outport
  Back Hip Pos [m m] : Outport  Port=2
  wires:
  Hip y/1 -> Mux1/2
  Mux1/1 -> Front Hip Pos [m m]/1
  Hip x/1 -> Mux1/1
  Hip y1/1 -> Mux2/2
  Mux2/1 -> Back Hip Pos [m m]/1
  Hip x1/1 -> Mux2/1
  CoM Pos [m m rad]/1 -> Hip x/1, Hip y/1, Hip y1/1, Hip x1/1

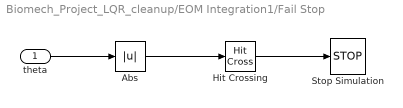
== system Biomech_Project_LQR_cleanup/EOM Integration1/Fail Stop ==
  theta : Inport
  Abs : Abs
  Hit Crossing : HitCross  HitCrossingOffset=1.57
  Stop Simulation : Stop
  wires:
  theta/1 -> Abs/1
  Hit Crossing/1 -> Stop Simulation/1
  Abs/1 -> Hit Crossing/1
